simulink library "EV_cooling"  (R2019b)
settings: Solver=VariableStepAuto  StartTime=0.0  StopTime=10.0  RelTol=1e-3
undefined symbols (not defined in the file): DiscIntNeverNeededParam
Description:
  | User defined library for EV
settings Model: Creator=francesco.mantuano  LastModifiedBy=francesco.mantuano

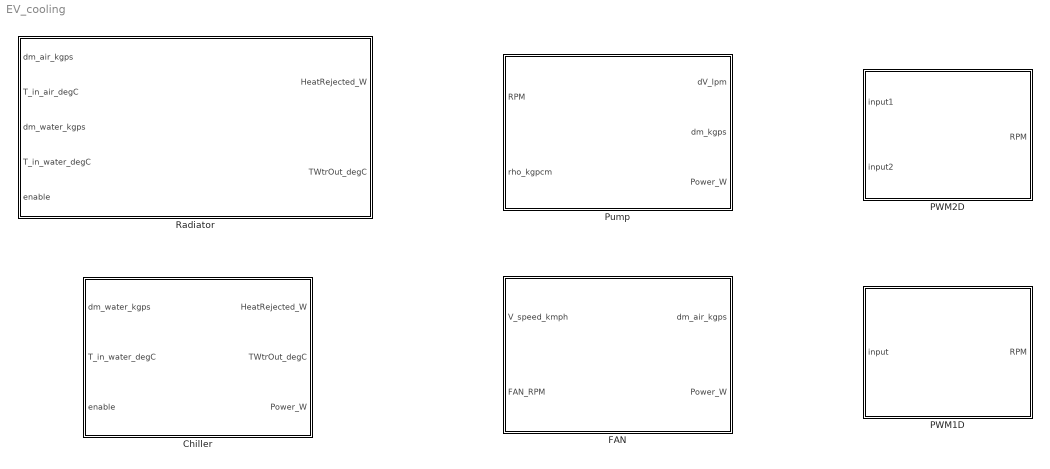
== system EV_cooling ==
  Chiller : Subsystem  mask(Chiller){dm_water_bp=0, T_water_bp=0, HR_map=0, COP=0}
      mask prompts: dm_water_bp "Water mass flow [kg/s] breakpoints"; T_water_bp "Water inlet temp [degC] breakpoints"; HR_map "Heat rejection map [W]"; COP "COP  [-]"
      mask help: The Chiller block outputs the Heat Rejected and the water outlet temperature.
      mask DialogControl Container2 Prompt: Inputs description
      mask DialogControl Control6 Prompt: - dm_water_kgps: the water mass flow [kg/s]
      mask DialogControl Control4 Prompt: - T_in_water_degC: water inlet temperature [degC]
      mask DialogControl Control8 Prompt: - enable: if 0 --> bypass (power = 0)
      mask DialogControl Container3 Prompt: Radiator parameters
      mask DialogControl Container5 Prompt: HeatRejection map
      mask DialogControl Container10 Prompt: Power consumption
  FAN : Subsystem  mask(FAN){speed_bp=0, RPM_bp=0, dm_map=0, power_map=0}
      mask prompts: speed_bp "vehicle speed [km/h] breakpoints"; RPM_bp "FAN RPM breakpoints"; dm_map "FAN mass flow [kg/s] map"; power_map "FAN power consumption [W] map"
      mask help:
      | The FAN block outputs the air mass flow and the power consumption.
      | Note that the maps are dependent on the Radiator - FAN couple
      mask DialogControl Container2 Prompt: Inputs description
      mask DialogControl Control3 Prompt: - V_speed_kmph: the actual vehicle speed [km/h]
      mask DialogControl Control2 Prompt: - FAN_RPM: the FAN actual RPMs [RPM]
      mask DialogControl Container3 Prompt: FAN parameters
  PWM1D : Subsystem  mask(PWM1D){input_bp=0, RPM_map=0}
      mask prompts: input_bp "Input breakpoints"; RPM_map "RPM map"
      mask help: The PWM block outputs the PWM controller [RPM].
      mask DialogControl Container2 Prompt: Inputs description
      mask DialogControl Control2 Prompt: - input: the control input
      mask DialogControl Container3 Prompt: PWM parameters
  PWM2D : Subsystem  mask(PWM2D){input1_bp=0, input2_bp=0, RPM_map=0}
      mask prompts: input1_bp "First input breakpoints"; input2_bp "Second input breakpoints"; RPM_map "RPM map"
      mask help: The PWM block outputs the PWM controller [RPM].
      mask DialogControl Container2 Prompt: Inputs description
      mask DialogControl Control2 Prompt: - input1: the first control input
      mask DialogControl Control3 Prompt: - input2: the second control input
      mask DialogControl Container3 Prompt: PWM parameters
  Pump : Subsystem  mask(Pump){RPM_bp=0, dV_map=0, power_map=0}
      mask prompts: RPM_bp "Pump RPM breakpoints"; dV_map "PUMP volumetric flow [lpm] map"; power_map "PUMP power consumption [W] map"
      mask help:
      | The Pump block outputs the volumetric and mass flow and the power consumption.
      | Note that the maps are dependent on the Pump - system couple (working point of the pump)
      mask DialogControl Container2 Prompt: Inputs description
      mask DialogControl Control2 Prompt: - RPM: the Pump actual RPMs [RPM]
      mask DialogControl Control3 Prompt: - rho_kgpcm: the liquid density [kg/cm]
      mask DialogControl Container3 Prompt: Pump parameters
  Radiator : Subsystem  mask(Radiator){dm_water_bp=0, dm_air_bp=0, normHR_map=0, FrontSurf=0}
      mask prompts: dm_water_bp "Water mass flow [kg/s] breakpoints"; dm_air_bp "Air mass flow [kg/s] breakpoints"; normHR_map "Heat rejection map [kW/(sm*K)]"; FrontSurf "Front Surface [sm] of the radiator"
      mask help: The Radiator block outputs the Heat Rejected and the water outlet temperature.
      mask DialogControl Container2 Prompt: Inputs description
      mask DialogControl DescTextVar Prompt: - dm_air_kgps: the air mass flow [kg/s]
      mask DialogControl Control3 Prompt: - T_in_air_degC: air inlet temperature [degC]
      mask DialogControl Control6 Prompt: - dm_water_kgps: the water mass flow [kg/s]
      mask DialogControl Control4 Prompt: - T_in_water_degC: water inlet temperature [degC]
      mask DialogControl Control8 Prompt: - enable: if 0 --> bypass
      mask DialogControl Container3 Prompt: Radiator parameters
      mask DialogControl Container5 Prompt: Normalized HeatRejection map
      mask DialogControl Container8 Prompt: Radiator Front Surface

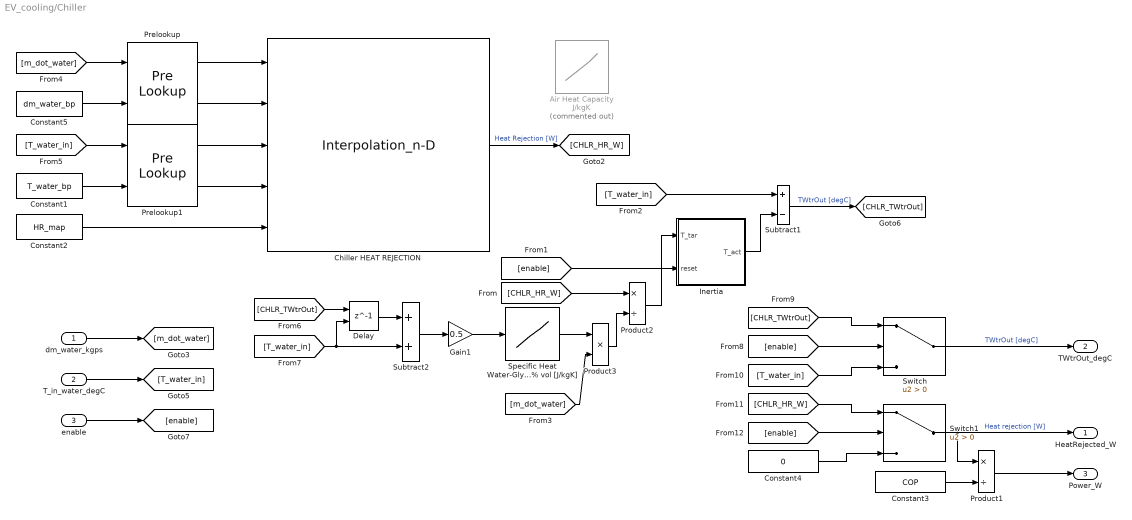
== system EV_cooling/Chiller ==
  dm_water_kgps : Inport
  T_in_water_degC : Inport  Port=2
  enable : Inport  Port=3
  Air Heat Capacity J/kgK : Lookup_n-D  Commented=on  NumberOfTableDimensions=1  BreakpointsForDimension1=[-40 -30 -20 -10 0 5 10 15 20 25 30 35 40 45 50 60 70 80 90 100]  Table=[1002 1004 1005 1006 1006 1007 1008 1009 1010 1011 1011 1012 1013 1014 1016 1017 1019 1020 1021 1022]  ExtrapMethod=Clip  RndMeth=Simplest  InputSameDT=on
  Chiller HEAT REJECTION : Interpolation_n-D  TableSource=Input port
      settings: InputPortMap=u0,u1,u2,u3,p2
  Constant1 : Constant  Value=T_water_bp
  Constant2 : Constant  Value=HR_map
  Constant3 : Constant  Value=COP
  Constant4 : Constant  Value=0
  Constant5 : Constant  Value=dm_water_bp
  Delay : Delay  DelayLength=1  InitialConditionSource=Input port
      settings: InputPortMap=u0,p4
  Gain1 : Gain  Gain=0.5
  Inertia : Subsystem
      mask help: Input the stationary temperature and output the actual temperature (due to thermal inertia)
  Prelookup : PreLookup  BreakpointsDataSource=Input port  BreakpointsData=[1:4]  FractionDataTypeStr=double
      settings: InputPortMap=u0,p1
  Prelookup1 : PreLookup  BreakpointsDataSource=Input port  BreakpointsData=[1:4]  FractionDataTypeStr=double
      settings: InputPortMap=u0,p1
  Product1 : Product  Inputs=*/
  Product2 : Product  Inputs=*/
  Product3 : Product
  Specific Heat Water-Glycol 80-20% vol [J/kgK] : Lookup_n-D  NumberOfTableDimensions=1  BreakpointsForDimension1=[-45.56 -17.78 10 37.77 65.55 93.33 121.11 148.88 176.66]  Table="[3841.6 3888.1  3934.6 3981.1 4027.6 4074.0 4120.5 4167.0 4213.6]"  ExtrapMethod=Clip  RndMeth=Simplest  InputSameDT=on
  Subtract1 : Sum  Inputs=+-
  Subtract2 : Sum
  Switch : Switch  Criteria=u2 > Threshold
  Switch1 : Switch  Criteria=u2 > Threshold
  HeatRejected_W : Outport
  TWtrOut_degC : Outport  Port=2
  Power_W : Outport  Port=3
  wires:
  Constant4/1 -> Switch1/3
  [CHLR_HR_W] -> Switch1/1
  Switch1/1 -> Product1/1, HeatRejected_W/1  "Heat rejection [W]"
  [enable] -> Switch1/2
  [T_water_in] -> Switch/3
  [CHLR_TWtrOut] -> Switch/1
  [enable] -> Switch/2
  enable/1 -> [enable]
  Constant2/1 -> Chiller HEAT REJECTION/5
  Subtract2/1 -> Gain1/1
  Chiller HEAT REJECTION/1 -> [CHLR_HR_W]  "Heat Rejection [W]"
  Prelookup/2 -> Chiller HEAT REJECTION/2
  T_in_water_degC/1 -> [T_water_in]
  Subtract1/1 -> [CHLR_TWtrOut]  "TWtrOut [degC]"
  [T_water_in] -> Subtract1/1
  Prelookup1/1 -> Chiller HEAT REJECTION/3
  Delay/1 -> Subtract2/1
  dm_water_kgps/1 -> [m_dot_water]
  Prelookup1/2 -> Chiller HEAT REJECTION/4
  [m_dot_water] -> Product3/2
  [T_water_in] -> Prelookup1/1
  Gain1/1 -> Specific Heat Water-Glycol 80-20% vol [J/kgK]/1
  Product3/1 -> Product2/2
  Prelookup/1 -> Chiller HEAT REJECTION/1
  Specific Heat Water-Glycol 80-20% vol [J/kgK]/1 -> Product3/1
  [T_water_in] -> Subtract2/2, Delay/2
  [CHLR_HR_W] -> Product2/1
  [CHLR_TWtrOut] -> Delay/1
  Constant1/1 -> Prelookup1/2
  [m_dot_water] -> Prelookup/1
  Constant5/1 -> Prelookup/2
  Product1/1 -> Power_W/1
  Constant3/1 -> Product1/2
  Switch/1 -> TWtrOut_degC/1  "TWtrOut [degC]"
  Inertia/1(T_act) -> Subtract1/2
  Product2/1 -> Inertia/1(T_tar)
  [enable] -> Inertia/2(reset)

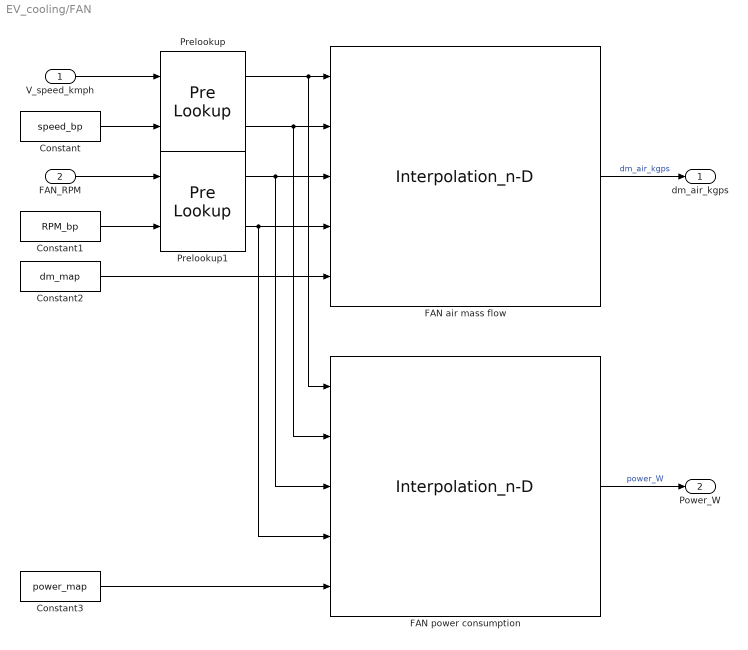
== system EV_cooling/FAN ==
  V_speed_kmph : Inport
  FAN_RPM : Inport  Port=2
  Constant : Constant  Value=speed_bp
  Constant1 : Constant  Value=RPM_bp
  Constant2 : Constant  Value=dm_map
  Constant3 : Constant  Value=power_map
  FAN air mass flow : Interpolation_n-D  TableSource=Input port
      settings: InputPortMap=u0,u1,u2,u3,p2
  FAN power consumption : Interpolation_n-D  TableSource=Input port
      settings: InputPortMap=u0,u1,u2,u3,p2
  Prelookup : PreLookup  BreakpointsDataSource=Input port  BreakpointsData=[1:4]  ExtrapMethod=Linear  FractionDataTypeStr=double
      settings: InputPortMap=u0,p1
  Prelookup1 : PreLookup  BreakpointsDataSource=Input port  BreakpointsData=[1:4]  ExtrapMethod=Linear  FractionDataTypeStr=double
      settings: InputPortMap=u0,p1
  dm_air_kgps : Outport
  Power_W : Outport  Port=2
  wires:
  Prelookup1/1 -> FAN power consumption/3, FAN air mass flow/3
  Prelookup1/2 -> FAN power consumption/4, FAN air mass flow/4
  Prelookup/1 -> FAN power consumption/1, FAN air mass flow/1
  Prelookup/2 -> FAN power consumption/2, FAN air mass flow/2
  FAN air mass flow/1 -> dm_air_kgps/1  "dm_air_kgps"
  V_speed_kmph/1 -> Prelookup/1
  FAN_RPM/1 -> Prelookup1/1
  FAN power consumption/1 -> Power_W/1  "power_W"
  Constant/1 -> Prelookup/2
  Constant1/1 -> Prelookup1/2
  Constant2/1 -> FAN air mass flow/5
  Constant3/1 -> FAN power consumption/5

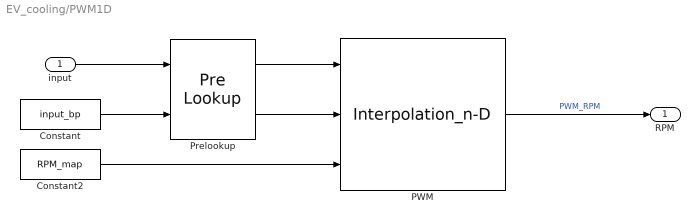
== system EV_cooling/PWM1D ==
  input : Inport
  Constant : Constant  Value=input_bp
  Constant2 : Constant  Value=RPM_map
  PWM : Interpolation_n-D  NumberOfTableDimensions=1  TableSource=Input port
      settings: InputPortMap=u0,u1,p2
  Prelookup : PreLookup  BreakpointsDataSource=Input port  BreakpointsData=[1:4]  ExtrapMethod=Linear  FractionDataTypeStr=double
      settings: InputPortMap=u0,p1
  RPM : Outport
  wires:
  Constant2/1 -> PWM/3
  Constant/1 -> Prelookup/2
  Prelookup/2 -> PWM/2
  Prelookup/1 -> PWM/1
  PWM/1 -> RPM/1  "PWM_RPM"
  input/1 -> Prelookup/1

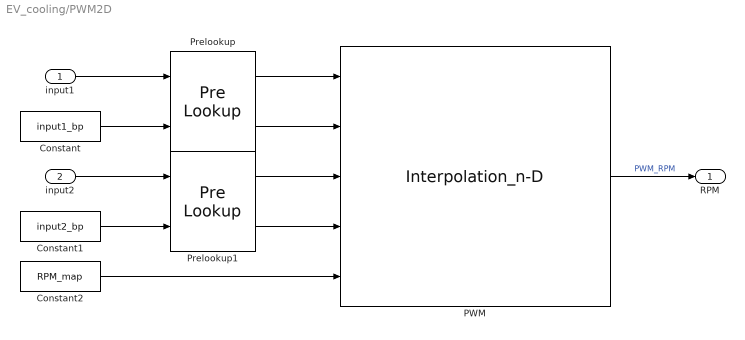
== system EV_cooling/PWM2D ==
  input1 : Inport
  input2 : Inport  Port=2
  Constant : Constant  Value=input1_bp
  Constant1 : Constant  Value=input2_bp
  Constant2 : Constant  Value=RPM_map
  PWM : Interpolation_n-D  TableSource=Input port
      settings: InputPortMap=u0,u1,u2,u3,p2
  Prelookup : PreLookup  BreakpointsDataSource=Input port  BreakpointsData=[1:4]  ExtrapMethod=Linear  FractionDataTypeStr=double
      settings: InputPortMap=u0,p1
  Prelookup1 : PreLookup  BreakpointsDataSource=Input port  BreakpointsData=[1:4]  FractionDataTypeStr=double
      settings: InputPortMap=u0,p1
  RPM : Outport
  wires:
  input1/1 -> Prelookup/1
  PWM/1 -> RPM/1  "PWM_RPM"
  Prelookup1/1 -> PWM/3
  Prelookup/1 -> PWM/1
  Prelookup/2 -> PWM/2
  Prelookup1/2 -> PWM/4
  input2/1 -> Prelookup1/1
  Constant/1 -> Prelookup/2
  Constant1/1 -> Prelookup1/2
  Constant2/1 -> PWM/5

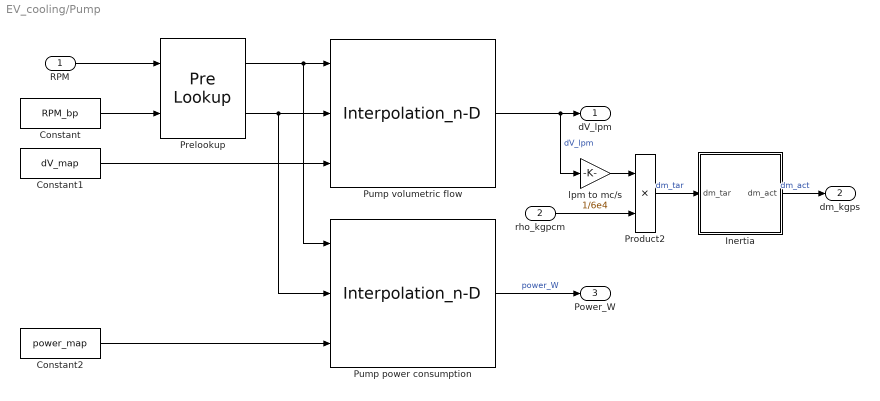
== system EV_cooling/Pump ==
  RPM : Inport
  rho_kgpcm : Inport  Port=2
  Constant : Constant  Value=RPM_bp
  Constant1 : Constant  Value=dV_map
  Constant2 : Constant  Value=power_map
  Inertia : Subsystem
      mask help: Input the target mass flow and output the actual mass flow (slower due to Inertia)
  Prelookup : PreLookup  BreakpointsDataSource=Input port  BreakpointsData=[1:4]  ExtrapMethod=Linear  FractionDataTypeStr=double
      settings: InputPortMap=u0,p1
  Product2 : Product
  Pump power consumption : Interpolation_n-D  NumberOfTableDimensions=1  TableSource=Input port
      settings: InputPortMap=u0,u1,p2
  Pump volumetric flow : Interpolation_n-D  NumberOfTableDimensions=1  TableSource=Input port
      settings: InputPortMap=u0,u1,p2
  lpm to mc/s : Gain  Gain=1/6e4
  dV_lpm : Outport
  dm_kgps : Outport  Port=2
  Power_W : Outport  Port=3
  wires:
  Prelookup/2 -> Pump power consumption/2, Pump volumetric flow/2
  Prelookup/1 -> Pump power consumption/1, Pump volumetric flow/1
  Pump volumetric flow/1 -> lpm to mc/s/1, dV_lpm/1  "dV_lpm"
  Pump power consumption/1 -> Power_W/1  "power_W"
  Product2/1 -> Inertia/1(dm_tar)  "dm_tar"
  lpm to mc/s/1 -> Product2/1
  RPM/1 -> Prelookup/1
  rho_kgpcm/1 -> Product2/2
  Inertia/1(dm_act) -> dm_kgps/1  "dm_act"
  Constant/1 -> Prelookup/2
  Constant1/1 -> Pump volumetric flow/3
  Constant2/1 -> Pump power consumption/3

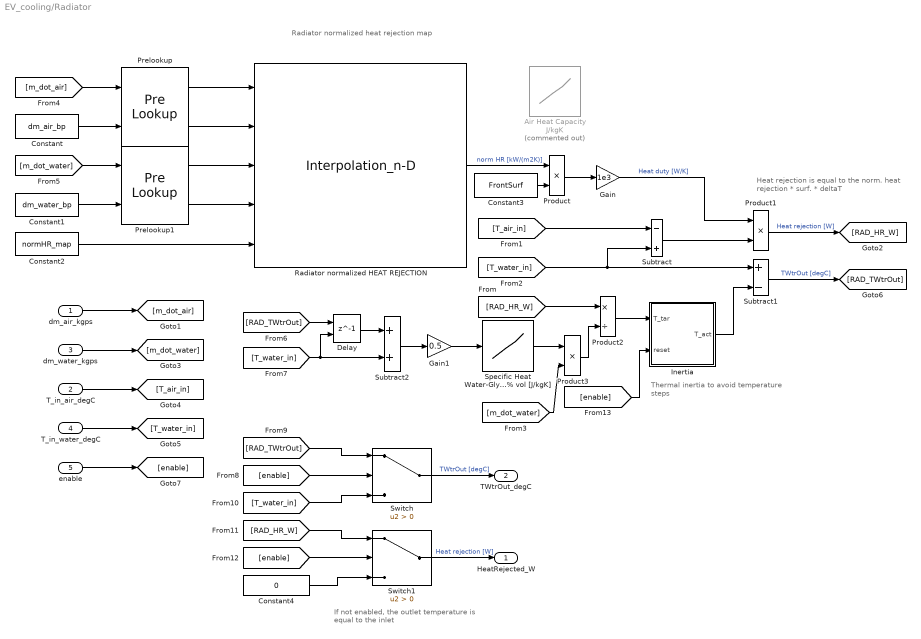
== system EV_cooling/Radiator ==
  note: Radiator normalized heat rejection map
  note: If not enabled, the outlet temperature is equal to the inlet
  note: Thermal inertia to avoid temperature steps
  note: Heat rejection is equal to the norm. heat rejection * surf. * deltaT
  dm_air_kgps : Inport
  T_in_air_degC : Inport  Port=2
  dm_water_kgps : Inport  Port=3
  T_in_water_degC : Inport  Port=4
  enable : Inport  Port=5
  Air Heat Capacity J/kgK : Lookup_n-D  Commented=on  NumberOfTableDimensions=1  BreakpointsForDimension1=[-40 -30 -20 -10 0 5 10 15 20 25 30 35 40 45 50 60 70 80 90 100]  Table=[1002 1004 1005 1006 1006 1007 1008 1009 1010 1011 1011 1012 1013 1014 1016 1017 1019 1020 1021 1022]  ExtrapMethod=Clip  RndMeth=Simplest  InputSameDT=on
  Constant : Constant  Value=dm_air_bp
  Constant1 : Constant  Value=dm_water_bp
  Constant2 : Constant  Value=normHR_map
  Constant3 : Constant  Value=FrontSurf
  Constant4 : Constant  Value=0
  Delay : Delay  DelayLength=1  InitialConditionSource=Input port
      settings: InputPortMap=u0,p4
  Gain : Gain  Gain=1e3
  Gain1 : Gain  Gain=0.5
  Inertia : Subsystem
      mask help: Input the stationary temperature and output the actual temperature (due to thermal inertia)
  Prelookup : PreLookup  BreakpointsDataSource=Input port  BreakpointsData=[1:4]  FractionDataTypeStr=double
      settings: InputPortMap=u0,p1
  Prelookup1 : PreLookup  BreakpointsDataSource=Input port  BreakpointsData=[1:4]  FractionDataTypeStr=double
      settings: InputPortMap=u0,p1
  Product : Product
  Product1 : Product
  Product2 : Product  Inputs=*/
  Product3 : Product
  Radiator normalized HEAT REJECTION : Interpolation_n-D  TableSource=Input port
      settings: InputPortMap=u0,u1,u2,u3,p2
  Specific Heat Water-Glycol 80-20% vol [J/kgK] : Lookup_n-D  NumberOfTableDimensions=1  BreakpointsForDimension1=[-45.56 -17.78 10 37.77 65.55 93.33 121.11 148.88 176.66]  Table="[3841.6 3888.1  3934.6 3981.1 4027.6 4074.0 4120.5 4167.0 4213.6]"  ExtrapMethod=Clip  RndMeth=Simplest  InputSameDT=on
  Subtract : Sum  Inputs=-+
  Subtract1 : Sum  Inputs=+-
  Subtract2 : Sum
  Switch : Switch  Criteria=u2 > Threshold
  Switch1 : Switch  Criteria=u2 > Threshold
  HeatRejected_W : Outport
  TWtrOut_degC : Outport  Port=2
  wires:
  Constant1/1 -> Prelookup1/2
  [RAD_TWtrOut] -> Delay/1
  [T_air_in] -> Subtract/1
  [RAD_HR_W] -> Product2/1
  Product/1 -> Gain/1
  [m_dot_air] -> Prelookup/1
  [T_water_in] -> Delay/2, Subtract2/2
  Specific Heat Water-Glycol 80-20% vol [J/kgK]/1 -> Product3/1
  Prelookup/1 -> Radiator normalized HEAT REJECTION/1
  Product3/1 -> Product2/2
  Gain1/1 -> Specific Heat Water-Glycol 80-20% vol [J/kgK]/1
  Product1/1 -> [RAD_HR_W]  "Heat rejection [W]"
  [m_dot_water] -> Prelookup1/1
  Subtract/1 -> Product1/2
  [m_dot_water] -> Product3/2
  Prelookup1/2 -> Radiator normalized HEAT REJECTION/4
  dm_water_kgps/1 -> [m_dot_water]
  Delay/1 -> Subtract2/1
  Prelookup1/1 -> Radiator normalized HEAT REJECTION/3
  [T_water_in] -> Subtract/2, Subtract1/1
  T_in_air_degC/1 -> [T_air_in]
  Subtract1/1 -> [RAD_TWtrOut]  "TWtrOut [degC]"
  T_in_water_degC/1 -> [T_water_in]
  Prelookup/2 -> Radiator normalized HEAT REJECTION/2
  Gain/1 -> Product1/1  "Heat duty [W/K]"
  Subtract2/1 -> Gain1/1
  Radiator normalized HEAT REJECTION/1 -> Product/1  "norm HR [kW/(m2K)]"
  dm_air_kgps/1 -> [m_dot_air]
  Constant/1 -> Prelookup/2
  Constant2/1 -> Radiator normalized HEAT REJECTION/5
  Constant3/1 -> Product/2
  enable/1 -> [enable]
  [enable] -> Switch/2
  Switch/1 -> TWtrOut_degC/1  "TWtrOut [degC]"
  [RAD_TWtrOut] -> Switch/1
  [T_water_in] -> Switch/3
  [enable] -> Switch1/2
  Switch1/1 -> HeatRejected_W/1  "Heat rejection [W]"
  [RAD_HR_W] -> Switch1/1
  Constant4/1 -> Switch1/3
  Product2/1 -> Inertia/1(T_tar)
  Inertia/1(T_act) -> Subtract1/2
  [enable] -> Inertia/2(reset)

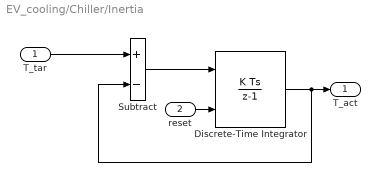
== system EV_cooling/Chiller/Inertia ==
  T_tar : Inport
  reset : Inport  Port=2
  Discrete-Time Integrator : DiscreteIntegrator  gainval=0.5  ExternalReset=either  SampleTime=-1  ICPrevOutput=DiscIntNeverNeededParam  ICPrevScaledInput=DiscIntNeverNeededParam
  Subtract : Sum  Inputs=+-
  T_act : Outport
  wires:
  T_tar/1 -> Subtract/1
  Subtract/1 -> Discrete-Time Integrator/1
  Discrete-Time Integrator/1 -> Subtract/2, T_act/1
  reset/1 -> Discrete-Time Integrator/2

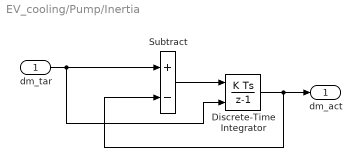
== system EV_cooling/Pump/Inertia ==
  dm_tar : Inport
  Discrete-Time Integrator : DiscreteIntegrator  gainval=0.8  InitialConditionSource=external  SampleTime=-1  ICPrevOutput=DiscIntNeverNeededParam  ICPrevScaledInput=DiscIntNeverNeededParam
  Subtract : Sum  Inputs=+-
  dm_act : Outport
  wires:
  dm_tar/1 -> Subtract/1, Discrete-Time Integrator/2
  Subtract/1 -> Discrete-Time Integrator/1
  Discrete-Time Integrator/1 -> Subtract/2, dm_act/1

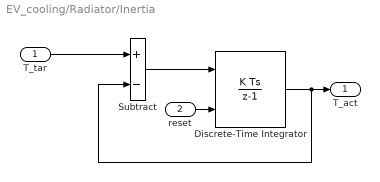
== system EV_cooling/Radiator/Inertia ==
  T_tar : Inport
  reset : Inport  Port=2
  Discrete-Time Integrator : DiscreteIntegrator  gainval=0.5  ExternalReset=either  SampleTime=-1  ICPrevOutput=DiscIntNeverNeededParam  ICPrevScaledInput=DiscIntNeverNeededParam
  Subtract : Sum  Inputs=+-
  T_act : Outport
  wires:
  T_tar/1 -> Subtract/1
  Subtract/1 -> Discrete-Time Integrator/1
  Discrete-Time Integrator/1 -> Subtract/2, T_act/1
  reset/1 -> Discrete-Time Integrator/2
